simulink model "q3_rbf_adaptive_controller_sim_at2019a"  (Simulink 9.3)
settings: Solver=VariableStepAuto  StartTime=0.0  StopTime=20  RelTol=1e-3
values from neighbouring files (symbols this model uses):
  alfa_1 = L*m*g/J    (= 14.7)    [q3_rbf_adaptive_controller_ws.m]
  alfa_2 = k*L^2/J    (= 1.5)    [q3_rbf_adaptive_controller_ws.m]
  alfa_3 = c*L^2/J    (= 1.5)    [q3_rbf_adaptive_controller_ws.m]
  B = [0; 1]    [q3_rbf_adaptive_controller_ws.m]
  b = (theta_max - theta_min)/n    (= 1.25663706144)    [q3_rbf_adaptive_controller_ws.m]
  c = [C1(:),C2(:)]'    [q3_rbf_adaptive_controller_ws.m]
  eta = 0.1    [q3_rbf_adaptive_controller_ws.m]
  gama = 40    [q3_rbf_adaptive_controller_ws.m]
  J = 2*(L^2/3)*m    (= 0.666666666667)    [q3_rbf_adaptive_controller_ws.m]
  kd = 10    [q3_rbf_adaptive_controller_ws.m]
  kp = 100    [q3_rbf_adaptive_controller_ws.m]
  m_min = 0.5    [q3_rbf_adaptive_controller_ws.m]
  P = lyap(A, Q)    [q3_rbf_adaptive_controller_ws.m]
  Ts = 0.001    [q3_rbf_adaptive_controller_ws.m]
  W0 = (rand(1, n^2) - 0.5)/10    [q3_rbf_adaptive_controller_ws.m]
libraries: simulink x1
settings Model: Creator=ronil  LastModifiedBy=ronil
settings DataIOCC: SaveFormat=Dataset  SignalLoggingSaveFormat=Dataset  ReturnWorkspaceOutputs=on
settings OptimizationCC: LifeSpan=auto
settings DebuggingCC: UnderspecifiedInitializationDetection=Simplified  MergeDetectMultiDrivingBlocksExec=error  FcnCallInpInsideContextMsg=error  SFUnexpectedBacktrackingDiag=error  SFNoUnconditionalDefaultTransitionDiag=error  SFExecutionAtInitializationDiag=warning  UnderSpecifiedDimensionMsg=error  ArithmeticOperatorsInVariantConditions=error
settings HardwareCC: ProdBitPerPointer=64  ProdBitPerSizeT=64  ProdBitPerPtrDiffT=64  ProdLargestAtomicFloat=Float  ProdIntDivRoundTo=Zero  ProdEndianess=LittleEndian  ProdWordSize=64  ProdHWDeviceType=Intel->x86-64 (Windows64)
settings ModelReferenceCC: PropagateSignalLabelsOutOfModel=on
settings SFSimCC: SimUseLocalCustomCode=on
settings RTWCC: RTWUseLocalCustomCode=on
settings CodeAppCC: StateflowObjectComments=off
settings GRTTargetCC: TargetLangStandard=C99 (ISO)  CombineOutputUpdateFcns=on  GRTInterface=off
settings ConfigComp: CovMetricSettings=dwe  CovHtmlReporting=off  CovSaveCumulativeToWorkspaceVar=off  CovSaveSingleToWorkspaceVar=off  CovExternalEMLEnable=on

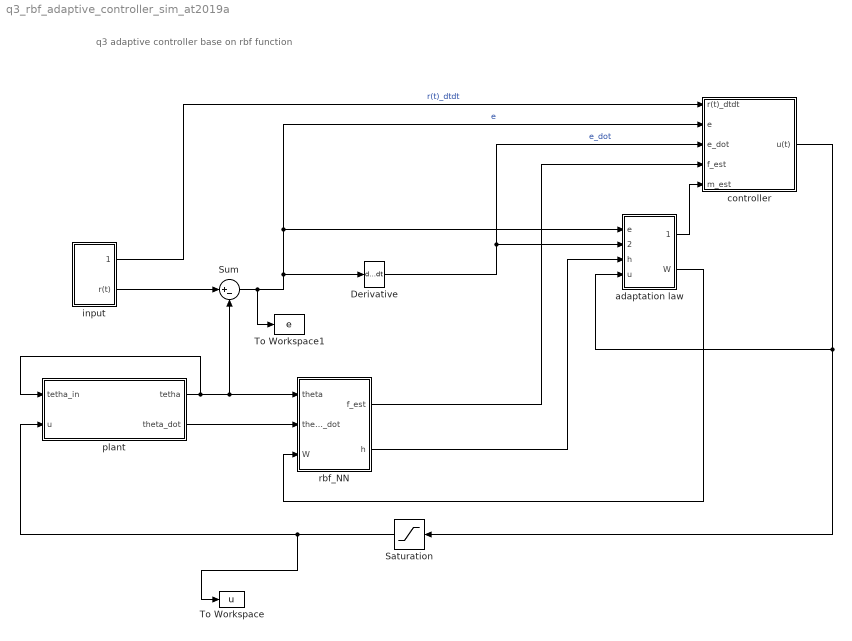
== system q3_rbf_adaptive_controller_sim_at2019a ==
  note: q3 adaptive controller base on rbf function
  Derivative : Derivative
  Saturation : Saturate  UpperLimit=1000  LowerLimit=-1000
  Sum : Sum  Inputs=|+-
  To Workspace : ToWorkspace  VariableName=u  SaveFormat=Timeseries  SampleTime=Ts
  To Workspace1 : ToWorkspace  VariableName=e  SaveFormat=Timeseries  SampleTime=Ts
  adaptation law : Subsystem
  controller : Subsystem
  input : Subsystem
  plant : Subsystem
  rbf_NN : Subsystem
  wires:
  input/2(r(t)) -> Sum/1
  Sum/1 -> controller/2(e), adaptation law/1(e), Derivative/1, To Workspace1/1  "e"
  Derivative/1 -> controller/3(e_dot), adaptation law/2(e_dot)  "e_dot"
  plant/1(tetha) -> plant/1(tetha_in), rbf_NN/1(theta), Sum/2
  Saturation/1 -> To Workspace/1, plant/2(u)
  adaptation law/2(W) -> rbf_NN/3(W)
  plant/2(theta_dot) -> rbf_NN/2(theta_dot)
  rbf_NN/2(h) -> adaptation law/3(h)
  controller/1(u(t)) -> Saturation/1, adaptation law/4(u)
  adaptation law/1(m_est) -> controller/5(m_est)
  input/1(r(t)_dtdt) -> controller/1(r(t)_dtdt)  "r(t)_dtdt"
  rbf_NN/1(f_est) -> controller/4(f_est)

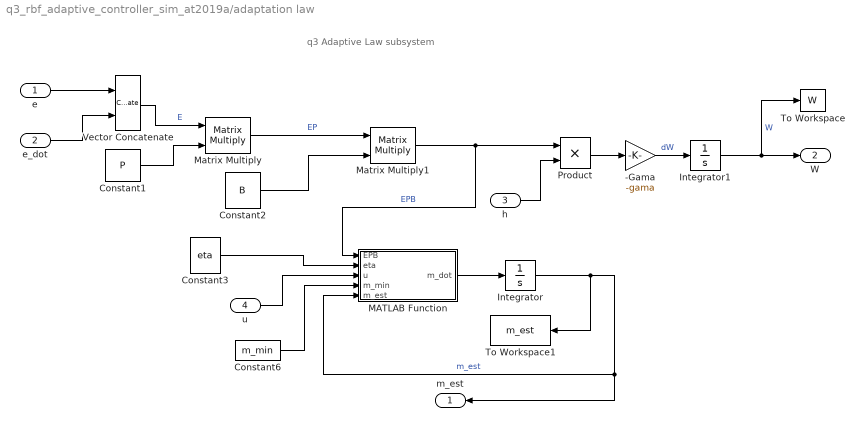
== system q3_rbf_adaptive_controller_sim_at2019a/adaptation law ==
  note: q3 Adaptive Law subsystem
  e : Inport
  e_dot : Inport  Port=2
  h : Inport  Port=3
  u : Inport  Port=4
  -Gama : Gain  Gain=-gama
  Constant1 : Constant  Value=P
  Constant2 : Constant  Value=B
  Constant3 : Constant  Value=eta
  Constant6 : Constant  Value=m_min
  Integrator : Integrator  InitialCondition=m_min
  Integrator1 : Integrator  InitialCondition=[W0]
  MATLAB Function : MATLAB Function  TreatAsAtomicUnit=on
  Matrix Multiply : Product  Multiplication=Matrix(*)
  Matrix Multiply1 : Product  Multiplication=Matrix(*)
  Product : Product
  To Workspace : ToWorkspace  VariableName=W  SaveFormat=Timeseries  SampleTime=Ts
      settings: Decimation=n
  To Workspace1 : ToWorkspace  VariableName=m_est  SaveFormat=Timeseries  SampleTime=Ts
  Vector Concatenate : Concatenate  Mode=Multidimensional array  ConcatenateDimension=2
  m_est : Outport
  W : Outport  Port=2
  wires:
  Integrator/1 -> MATLAB Function/5(m_est), m_est/1, To Workspace1/1  "m_est"
  MATLAB Function/1(m_dot) -> Integrator/1
  Constant3/1 -> MATLAB Function/2(eta)
  Constant6/1 -> MATLAB Function/4(m_min)
  u/1 -> MATLAB Function/3(u)
  -Gama/1 -> Integrator1/1  "dW"
  Product/1 -> -Gama/1
  e_dot/1 -> Vector Concatenate/2
  h/1 -> Product/2
  Matrix Multiply1/1 -> Product/1, MATLAB Function/1(EPB)  "EPB"
  Constant2/1 -> Matrix Multiply1/2
  Matrix Multiply/1 -> Matrix Multiply1/1  "EP"
  Vector Concatenate/1 -> Matrix Multiply/1  "E"
  Constant1/1 -> Matrix Multiply/2
  e/1 -> Vector Concatenate/1
  Integrator1/1 -> W/1, To Workspace/1  "W"

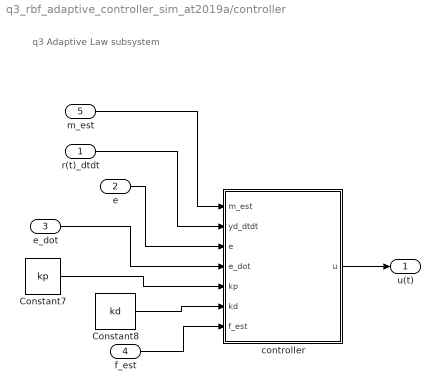
== system q3_rbf_adaptive_controller_sim_at2019a/controller ==
  note: q3 Adaptive Law subsystem
  r(t)_dtdt : Inport
  e : Inport  Port=2
  e_dot : Inport  Port=3
  f_est : Inport  Port=4
  m_est : Inport  Port=5
  Constant7 : Constant  Value=kp
  Constant8 : Constant  Value=kd
  controller : MATLAB Function  TreatAsAtomicUnit=on
  u(t) : Outport
  wires:
  Constant8/1 -> controller/6(kd)
  r(t)_dtdt/1 -> controller/2(yd_dtdt)
  e/1 -> controller/3(e)
  Constant7/1 -> controller/5(kp)
  f_est/1 -> controller/7(f_est)
  controller/1(u) -> u(t)/1
  m_est/1 -> controller/1(m_est)
  e_dot/1 -> controller/4(e_dot)

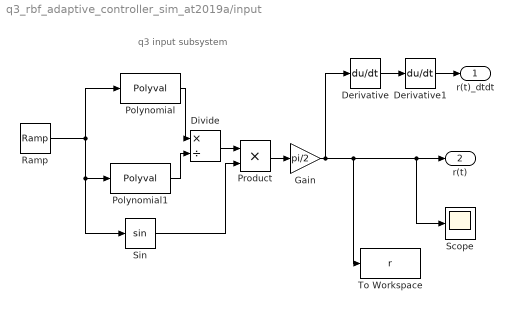
== system q3_rbf_adaptive_controller_sim_at2019a/input ==
  note: q3 input subsystem
  Derivative : Derivative
  Derivative1 : Derivative
  Divide : Product  Inputs=*/
  Gain : Gain  Gain=pi/2
  Polynomial : Polyval  Coefs=[1 0 0 0 0 0]
  Polynomial1 : Polyval  Coefs=[1 0 0 0 0 1000]
  Product : Product
  Ramp : simulink/Sources/Ramp  slope=1  start=0  InitialOutput=0  VectorParams1D=off
  Scope : Scope
  Sin : Trigonometry
  To Workspace : ToWorkspace  VariableName=r  SaveFormat=Timeseries  SampleTime=Ts
  r(t)_dtdt : Outport
  r(t) : Outport  Port=2
  wires:
  Ramp/1 -> Polynomial/1, Sin/1, Polynomial1/1
  Polynomial1/1 -> Divide/2
  Gain/1 -> Derivative/1, To Workspace/1, Scope/1, r(t)/1
  Polynomial/1 -> Divide/1
  Derivative/1 -> Derivative1/1
  Derivative1/1 -> r(t)_dtdt/1
  Divide/1 -> Product/1
  Sin/1 -> Product/2
  Product/1 -> Gain/1

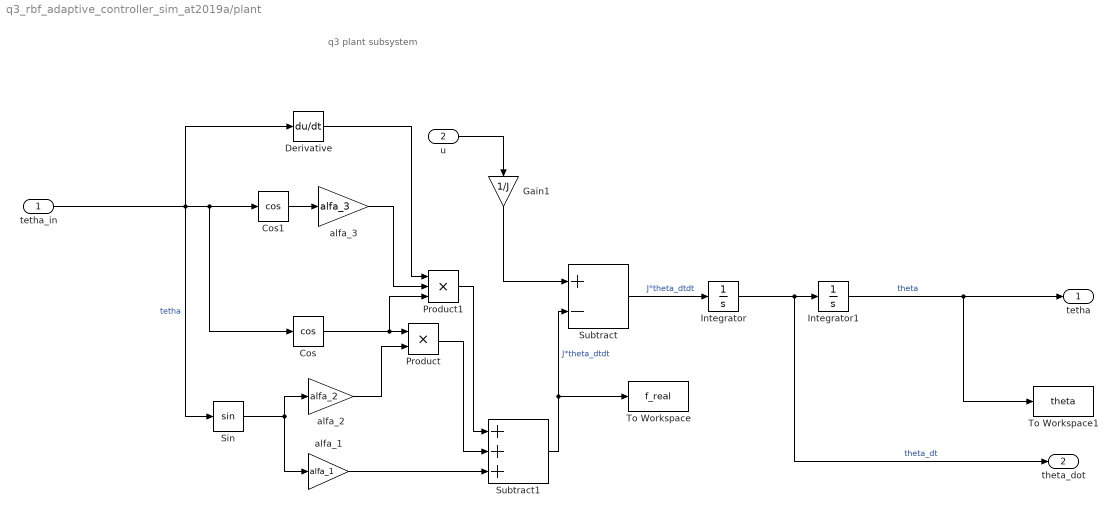
== system q3_rbf_adaptive_controller_sim_at2019a/plant ==
  note: q3 plant subsystem
  tetha_in : Inport
  u : Inport  Port=2
  Cos : Trigonometry  Operator=cos
  Cos1 : Trigonometry  Operator=cos
  Derivative : Derivative
  Gain1 : Gain  Gain=1/J
  Integrator : Integrator
  Integrator1 : Integrator
  Product : Product
  Product1 : Product  Inputs=3
  Sin : Trigonometry
  Subtract : Sum  Inputs=+-
  Subtract1 : Sum  Inputs=+++
  To Workspace : ToWorkspace  VariableName=f_real  SaveFormat=Timeseries  SampleTime=Ts
  To Workspace1 : ToWorkspace  VariableName=theta  SaveFormat=Timeseries  SampleTime=Ts
  alfa_1 : Gain  Gain=alfa_1
  alfa_2 : Gain  Gain=alfa_2
  alfa_3 : Gain  Gain=alfa_3
  tetha : Outport
  theta_dot : Outport  Port=2
  wires:
  Integrator1/1 -> To Workspace1/1, tetha/1  "theta"
  alfa_1/1 -> Subtract1/3
  Integrator/1 -> theta_dot/1, Integrator1/1  "theta_dt"
  Product/1 -> Subtract1/2
  u/1 -> Gain1/1
  tetha_in/1 -> Derivative/1, Sin/1, Cos/1, Cos1/1  "tetha"
  alfa_3/1 -> Product1/2
  alfa_2/1 -> Product/2
  Subtract/1 -> Integrator/1  "J*theta_dtdt"
  Cos1/1 -> alfa_3/1
  Derivative/1 -> Product1/1
  Product1/1 -> Subtract1/1
  Gain1/1 -> Subtract/1
  Cos/1 -> Product1/3, Product/1
  Sin/1 -> alfa_2/1, alfa_1/1
  Subtract1/1 -> To Workspace/1, Subtract/2  "J*theta_dtdt"

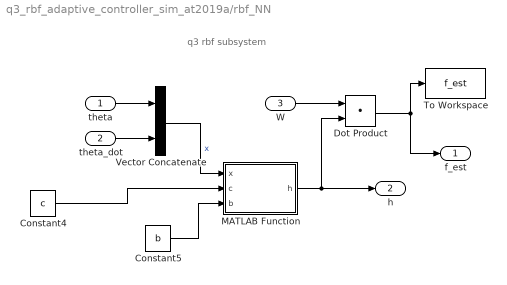
== system q3_rbf_adaptive_controller_sim_at2019a/rbf_NN ==
  note: q3 rbf subsystem
  theta : Inport
  theta_dot : Inport  Port=2
  W : Inport  Port=3
  Constant4 : Constant  Value=c
  Constant5 : Constant  Value=b
  Dot Product : DotProduct  InputSameDT=on  OutDataTypeStr=Inherit: Inherit via internal rule
  MATLAB Function : MATLAB Function  TreatAsAtomicUnit=on
  To Workspace : ToWorkspace  VariableName=f_est  SaveFormat=Timeseries  SampleTime=Ts
  Vector Concatenate : Concatenate
  f_est : Outport
  h : Outport  Port=2
  wires:
  MATLAB Function/1(h) -> Dot Product/2, h/1
  Dot Product/1 -> f_est/1, To Workspace/1
  W/1 -> Dot Product/1
  Constant5/1 -> MATLAB Function/3(b)
  Constant4/1 -> MATLAB Function/2(c)
  Vector Concatenate/1 -> MATLAB Function/1(x)  "x"
  theta_dot/1 -> Vector Concatenate/2
  theta/1 -> Vector Concatenate/1

== matlab function controller/controller ==
  data: m_est input double; yd_dtdt input double; e input double; e_dot input double; kp input double; kd input double; f_est input double; u output double
function u = controller(m_est,yd_dtdt,e,e_dot,kp,kd, f_est)
u = 1/m_est*(-f_est+yd_dtdt+kp*e+kd*e_dot);
end

== matlab function rbf_NN/MATLAB Function ==
  data: x input double; h output double; c input double; b input double
function h = fcn(x, c, b)
m=length(c(1,:));
h = zeros(m,1);
for j=1:m
    h(j)=exp(-norm(x-c(:,j))^2/(2*b^2));
end

== matlab function adaptation law/MATLAB Function ==
  data: EPB input double; eta input double; u input double; m_min input double; m_est input double; m_dot output double
function m_dot = func1(EPB,eta, u, m_min, m_est)
a = EPB*u;
if a > 0
    m_dot = eta.*a;
else
    if m_est>m_min
         m_dot = eta.*a;
    else
        m_dot = 1/eta;
    end
end
